simulink model "eg_8_05_R2018a"  (R2018a)
settings: Solver=ode4  StartTime=0.0  StopTime=10  FixedStep=0.001  RelTol=1e-3  EnableMultiTasking=on
values from neighbouring files (symbols this model uses):
  A = [  0   1 ... (first row only)    [eg_8_01.m]    (also in eg_8_02_1a.m; eg_8_02_1b.m; eg_8_02_1c.m; eg_8_02_1d.m)
  B = [ 0 ... (first row only)    [eg_8_01.m]    (also in eg_8_02_1a.m; eg_8_02_1b.m; eg_8_02_1c.m; eg_8_02_1d.m)
  C = [ 0  0  1  0 ]    [eg_8_05.m]
  Fa = [ -K+2*G*inv(P22)*P12'  1 ]*inv(M0)*[ zeros(n,p) ... (first row only)    [eg_8_05.m]
  Fb = - 2*G*inv(P22)*P12'    [eg_8_05.m]
  G = - inv(Re)*B'*P12    [eg_8_05.m]
  K = [ 5  -1 ]    [eg_8_01.m]    (also in eg_8_02_1a.m = - lqr(A,B,Q,R); eg_8_02_1b.m = double(K); eg_8_02_1c.m = - inv(R)*B'*P; eg_8_02_1d.m = - lqr(A,B,Q,R))
  x0 = [ 1 ... (first row only)    [eg_8_01.m]    (also in eg_8_02_1b.m; eg_8_02_1c.m; eg_8_02_1d.m; eg_8_02_2b.m)
settings Model: Creator=kawata  LastModifiedBy=kawata
settings DataIOCC: LimitDataPoints=on  SaveFormat=Array  SignalLoggingSaveFormat=ModelDataLogs  SignalLoggingName=sigsOut
settings OptimizationCC: ExpressionDepthLimit=2147483647  InitFltsAndDblsToZero=on  LifeSpan=inf
settings DebuggingCC: SaveWithParameterizedLinksMsg=none  UnderspecifiedInitializationDetection=Classic  MergeDetectMultiDrivingBlocksExec=none  SignalResolutionControl=TryResolveAllWithWarning  MultiTaskDSMMsg=warning  MultiTaskCondExecSysMsg=none  FcnCallInpInsideContextMsg=warning  StateNameClashWarn=warning  SFUnexpectedBacktrackingDiag=warning  SFNoUnconditionalDefaultTransitionDiag=warning  SFExecutionAtInitializationDiag=none
settings HardwareCC: ProdBitPerPointer=32  ProdBitPerSizeT=32  ProdBitPerPtrDiffT=32  ProdLargestAtomicFloat=None  ProdIntDivRoundTo=Undefined  ProdEndianess=Unspecified  ProdWordSize=32  ProdHWDeviceType=32-bit Generic  TargetUnknown=on
settings ModelReferenceCC: PropagateSignalLabelsOutOfModel=off
settings CodeAppCC: StateflowObjectComments=on
settings GRTTargetCC: TargetLangStandard=C89/C90 (ANSI)  GeneratePreprocessorConditionals=Disable all  CombineOutputUpdateFcns=off  GRTInterface=on
settings ConfigComp: CovMetricSettings=dw  CovHtmlReporting=on  CovSaveCumulativeToWorkspaceVar=on  CovSaveSingleToWorkspaceVar=on  CovExternalEMLEnable=off

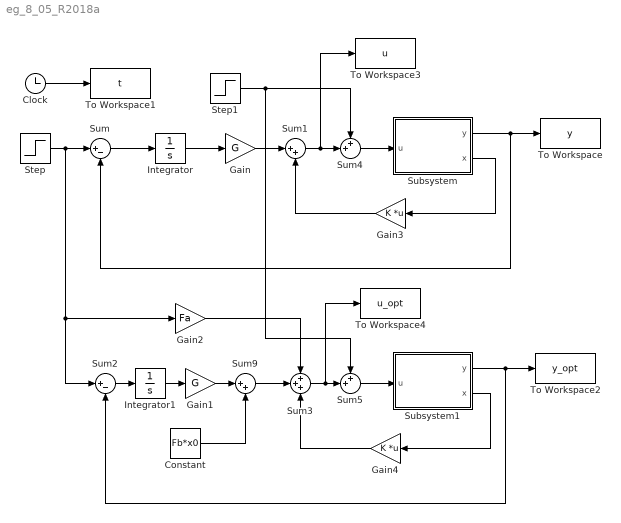
== system eg_8_05_R2018a ==
  Clock : Clock
  Constant : Constant  Value=Fb*x0
  Gain : Gain  Gain=G  SaturateOnIntegerOverflow=on  OutDataTypeStr=Inherit: Same as input  ParamDataTypeStr=Inherit: Same as input
  Gain1 : Gain  Gain=G  SaturateOnIntegerOverflow=on  OutDataTypeStr=Inherit: Same as input  ParamDataTypeStr=Inherit: Same as input
  Gain2 : Gain  Gain=Fa  SaturateOnIntegerOverflow=on  OutDataTypeStr=Inherit: Same as input  ParamDataTypeStr=Inherit: Same as input
  Gain3 : Gain  Gain=K  Multiplication=Matrix(K*u)  SaturateOnIntegerOverflow=on  OutDataTypeStr=Inherit: Same as input  ParamDataTypeStr=Inherit: Same as input
  Gain4 : Gain  Gain=K  Multiplication=Matrix(K*u)  SaturateOnIntegerOverflow=on  OutDataTypeStr=Inherit: Same as input  ParamDataTypeStr=Inherit: Same as input
  Integrator : Integrator
  Integrator1 : Integrator
  Step : Step  Time=0  SampleTime=0
  Step1 : Step  Time=5  SampleTime=0
  Subsystem : Subsystem
  Subsystem1 : Subsystem
  Sum : Sum  Inputs=|+-  SaturateOnIntegerOverflow=on  InputSameDT=on  OutDataTypeStr=Inherit: Same as first input
  Sum1 : Sum  Inputs=|++  SaturateOnIntegerOverflow=on  InputSameDT=on  OutDataTypeStr=Inherit: Same as first input
  Sum2 : Sum  Inputs=|+-  SaturateOnIntegerOverflow=on  InputSameDT=on  OutDataTypeStr=Inherit: Same as first input
  Sum3 : Sum  Inputs=+++  SaturateOnIntegerOverflow=on  InputSameDT=on  OutDataTypeStr=Inherit: Same as first input
  Sum4 : Sum  Inputs=++|  SaturateOnIntegerOverflow=on  InputSameDT=on  OutDataTypeStr=Inherit: Same as first input
  Sum5 : Sum  Inputs=++|  SaturateOnIntegerOverflow=on  InputSameDT=on  OutDataTypeStr=Inherit: Same as first input
  Sum9 : Sum  Inputs=|++  SaturateOnIntegerOverflow=on  InputSameDT=on  OutDataTypeStr=Inherit: Same as first input
  To Workspace : ToWorkspace  VariableName=y  SampleTime=-1
  To Workspace1 : ToWorkspace  VariableName=t  SampleTime=-1
  To Workspace2 : ToWorkspace  VariableName=y_opt  SampleTime=-1
  To Workspace3 : ToWorkspace  VariableName=u  SampleTime=-1
  To Workspace4 : ToWorkspace  VariableName=u_opt  SampleTime=-1
  wires:
  Subsystem/1(y) -> To Workspace/1, Sum/2
  Subsystem/2(x) -> Gain3/1
  Clock/1 -> To Workspace1/1
  Step1/1 -> Sum4/1, Sum5/1
  Gain3/1 -> Sum1/2
  Step/1 -> Sum/1, Gain2/1, Sum2/1
  Sum/1 -> Integrator/1
  Integrator/1 -> Gain/1
  Subsystem1/1(y) -> Sum2/2, To Workspace2/1
  Subsystem1/2(x) -> Gain4/1
  Sum2/1 -> Integrator1/1
  Gain4/1 -> Sum3/3
  Sum5/1 -> Subsystem1/1(u)
  Sum3/1 -> Sum5/2, To Workspace4/1
  Gain2/1 -> Sum3/1
  Gain/1 -> Sum1/1
  Sum1/1 -> Sum4/2, To Workspace3/1
  Sum4/1 -> Subsystem/1(u)
  Constant/1 -> Sum9/2
  Integrator1/1 -> Gain1/1
  Gain1/1 -> Sum9/1
  Sum9/1 -> Sum3/2

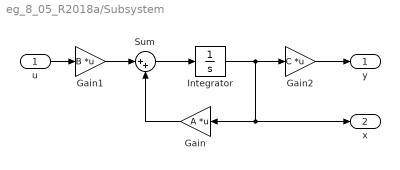
== system eg_8_05_R2018a/Subsystem ==
  u : Inport
  Gain : Gain  Gain=A  Multiplication=Matrix(K*u)  SaturateOnIntegerOverflow=on  OutDataTypeStr=Inherit: Same as input  ParamDataTypeStr=Inherit: Same as input
  Gain1 : Gain  Gain=B  Multiplication=Matrix(K*u)  SaturateOnIntegerOverflow=on  OutDataTypeStr=Inherit: Same as input  ParamDataTypeStr=Inherit: Same as input
  Gain2 : Gain  Gain=C  Multiplication=Matrix(K*u)  SaturateOnIntegerOverflow=on  OutDataTypeStr=Inherit: Same as input  ParamDataTypeStr=Inherit: Same as input
  Integrator : Integrator  InitialCondition=x0
  Sum : Sum  Inputs=|++  SaturateOnIntegerOverflow=on  InputSameDT=on  OutDataTypeStr=Inherit: Same as first input
  y : Outport
  x : Outport  Port=2
  wires:
  Gain/1 -> Sum/2
  Sum/1 -> Integrator/1
  Gain1/1 -> Sum/1
  Integrator/1 -> Gain2/1, Gain/1, x/1
  u/1 -> Gain1/1
  Gain2/1 -> y/1

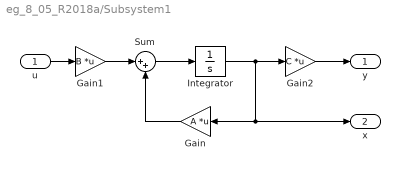
== system eg_8_05_R2018a/Subsystem1 ==
  u : Inport
  Gain : Gain  Gain=A  Multiplication=Matrix(K*u)  SaturateOnIntegerOverflow=on  OutDataTypeStr=Inherit: Same as input  ParamDataTypeStr=Inherit: Same as input
  Gain1 : Gain  Gain=B  Multiplication=Matrix(K*u)  SaturateOnIntegerOverflow=on  OutDataTypeStr=Inherit: Same as input  ParamDataTypeStr=Inherit: Same as input
  Gain2 : Gain  Gain=C  Multiplication=Matrix(K*u)  SaturateOnIntegerOverflow=on  OutDataTypeStr=Inherit: Same as input  ParamDataTypeStr=Inherit: Same as input
  Integrator : Integrator  InitialCondition=x0
  Sum : Sum  Inputs=|++  SaturateOnIntegerOverflow=on  InputSameDT=on  OutDataTypeStr=Inherit: Same as first input
  y : Outport
  x : Outport  Port=2
  wires:
  Gain/1 -> Sum/2
  Sum/1 -> Integrator/1
  Gain1/1 -> Sum/1
  Integrator/1 -> Gain2/1, Gain/1, x/1
  u/1 -> Gain1/1
  Gain2/1 -> y/1
